simulink model "bell_nexus_4ex_model"  (R2024a)
settings: Solver=ode4  StartTime=0.0  StopTime=simt  FixedStep=st  RelTol=1e-3
values from neighbouring files (symbols this model uses):
  ailer_lim = [-15 20]    [bell_nexus_4ex_params.m]
  B_lat_ext = [B_lat, Bw_lat]    [bell_nexus_4ex.m]
  B_lon_ext = [B_lon, Bw_lon]    [bell_nexus_4ex.m]
  C_lat_ext = [C_lat; eye(1,4)]    [bell_nexus_4ex.m]
  C_lon_ext = [C_lon; eye(2,4)]    [bell_nexus_4ex.m]
  D_lat_ext = blkdiag(D_lat, Tw_lat(1,:))    [bell_nexus_4ex.m]
  D_lon_ext = blkdiag(D_lon, Tw_lon(1:2,:))    [bell_nexus_4ex.m]
  deriv_lag = 0.005    [bell_nexus_4ex.m]    (also in bell_nexus_4ex_params.m = 0.05)
  elev_lim = [-15 22]    [bell_nexus_4ex_params.m]
  elev_pf_tau = 0.7    [bell_nexus_4ex_params.m]
  kd_rudder = 0    [bell_nexus_4ex_params.m]
  ki_rudder = 0    [bell_nexus_4ex_params.m]
  kp_rudder = 0.5    [bell_nexus_4ex_params.m]
  phi_slope = 0    [bell_nexus_4ex.m]
  phi_sp = 0    [bell_nexus_4ex.m]
  phi_st_time = 4    [bell_nexus_4ex.m]
  r_slope = 0    [bell_nexus_4ex.m]
  r_sp = 0    [bell_nexus_4ex.m]
  r_st_time = 4    [bell_nexus_4ex.m]
  rate_lim = 30    [bell_nexus_4ex_params.m]
  rudder_lim = [-25 25]    [bell_nexus_4ex_params.m]
  tau = 0.1    [bell_nexus_4ex_params.m]
  theta_slope = 0    [bell_nexus_4ex.m]
  theta_sp = 0    [bell_nexus_4ex.m]
  theta_st_time = 4    [bell_nexus_4ex.m]
  w_st_time = 4    [bell_nexus_4ex.m]
  wind_lat = [0 0 0]    [bell_nexus_4ex.m]
  wind_lon = [0 0 0]    [bell_nexus_4ex.m]
undefined symbols (not defined in the file or in its folder): A_lat, A_lon, kd_aileron, kd_elevator, ki_aileron, ki_elevator, kp_aileron, kp_elevator, u0
libraries: slpidlib x3, simulink x3
settings Model: Creator=pries  LastModifiedBy=pries
settings RTWCC: GPUComputeCapability=3.5

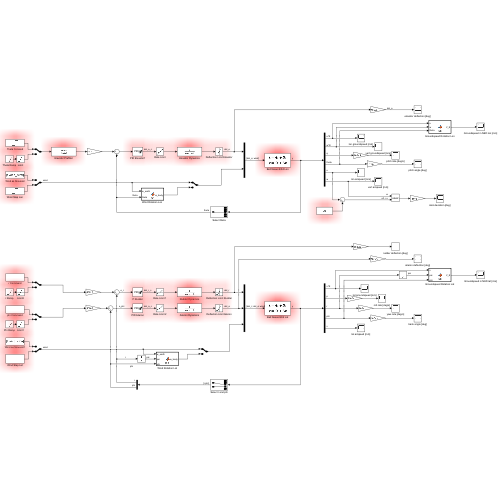
[thumbnail: Simulink's stored preview of the top-level diagram]
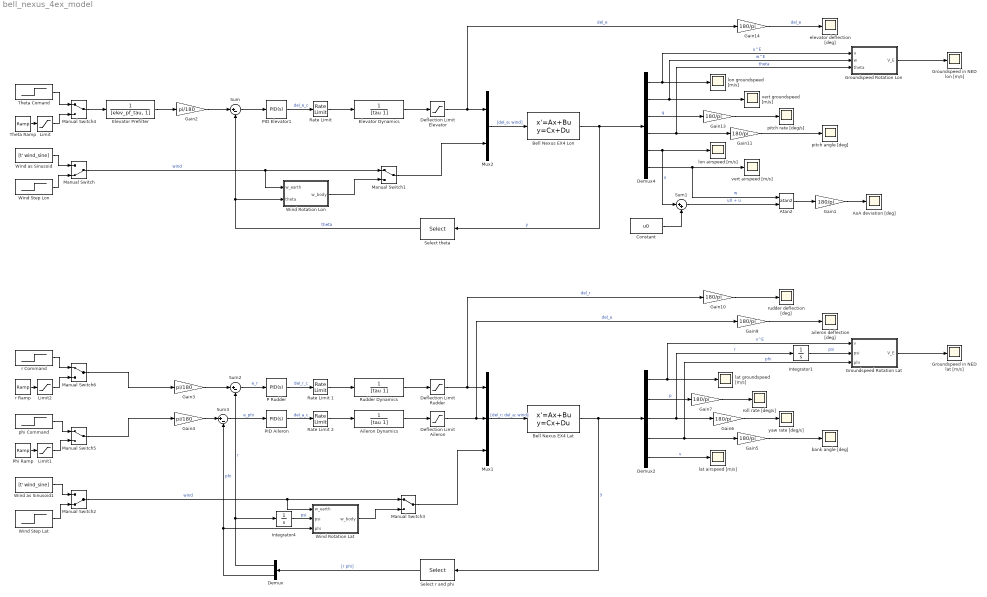
== system bell_nexus_4ex_model ==
  Aileron Dynamics : TransferFcn  Denominator=[tau 1]
  AoA deviation [deg] : Scope
  Atan2 : Trigonometry  Operator=atan2
  Bell Nexus EX4 Lat : StateSpace  A=A_lat  B=B_lat_ext  C=C_lat_ext  D=D_lat_ext  InitialCondition=0  ParameterTunability=Optimized
  Bell Nexus EX4 Lon : StateSpace  A=A_lon  B=B_lon_ext  C=C_lon_ext  D=D_lon_ext  InitialCondition=0
  Constant : Constant  Value=u0
  Deflection Limit Aileron : Saturate  UpperLimit=ailer_lim(2)*pi/180  LowerLimit=ailer_lim(1)*pi/180
  Deflection Limit Elevator : Saturate  UpperLimit=elev_lim(2)*pi/180  LowerLimit=elev_lim(1)*pi/180
  Deflection Limit Rudder : Saturate  UpperLimit=rudder_lim(2)*pi/180  LowerLimit=rudder_lim(1)*pi/180
  Demux : Demux  Outputs=2
  Demux2 : Demux  Outputs=5
  Demux4 : Demux  Outputs=6
  Elevator Dynamics : TransferFcn  Denominator=[tau 1]
  Elevator Prefilter : TransferFcn  Denominator=[elev_pf_tau, 1]
  Gain{1,5..7,9..11,13..14} (9 alike) : Gain  Gain=180/pi
  Gain2 : Gain  Gain=pi/180
  Gain3 : Gain  Gain=pi/180
  Gain4 : Gain  Gain=pi/180
  Groundspeed Rotation Lat : MATLAB Function  TreatAsAtomicUnit=on
  Groundspeed Rotation Lon : MATLAB Function  TreatAsAtomicUnit=on
  Groundspeed in NED lat [m/s] : Scope
  Groundspeed in NED lon [m/s] : Scope
  Integrator1 : Integrator
  Integrator4 : Integrator
  Limit : Saturate  UpperLimit=abs(theta_sp)  LowerLimit=-abs(theta_sp)
  Limit1 : Saturate  UpperLimit=abs(phi_sp)  LowerLimit=-abs(phi_sp)  LinearizeAsGain=off
  Limit2 : Saturate  UpperLimit=abs(r_sp)  LowerLimit=-abs(r_sp)  LinearizeAsGain=off
  Manual Switch : ManualSwitch  CurrentSetting=0
  Manual Switch{1,3..6} (5 alike) : ManualSwitch
  Manual Switch2 : ManualSwitch  CurrentSetting=0
  Mux1 : Mux  Inputs=3
  Mux2 : Mux  Inputs=2
  P Rudder : slpidlib/PID Controller  Controller=PID  Form=Parallel  TimeDomain=Continuous-time  UseExternalTs=off  SampleTime=-1  IntegratorMethod=Forward Euler  FilterMethod=Forward Euler  ControllerParametersSource=internal  P=kp_rudder  I=ki_rudder  UseKiTs=off  D=kd_rudder  UseExternalDerivativeSource=off  N=1/deriv_lag  UseFilter=on  TunerSelectOption=Transfer Function Based (PID Tuner App)  InitialConditionSource=internal  InitialConditionForIntegrator=0  InitialConditionForFilter=0  DifferentiatorICPrevScaledInput=0  ExternalReset=none  TrackingMode=off  Kt=1  LimitOutput=on  SatLimitsSource=internal  UpperSaturationLimit=rudder_lim(2)*pi/180  LowerSaturationLimit=rudder_lim(1)*pi/180  LinearizeAsGain=on  AntiWindupMode=back-calculation  Kb=1  LimitIntegrator=off  UpperIntegratorSaturationLimit=inf  LowerIntegratorSaturationLimit=-inf  POutMin=[]  POutMax=[]  IOutMin=[]  IOutMax=[]  DOutMin=[]  DOutMax=[]  NOutMin=[]  NOutMax=[]  SumOutMin=[]  SumOutMax=[]  SaturationOutMin=[]  SaturationOutMax=[]  PParamMin=[]  PParamMax=[]  IParamMin=[]  IParamMax=[]  DParamMin=[]  DParamMax=[]  NParamMin=[]  NParamMax=[]  KbParamMin=[]  KbParamMax=[]  KtParamMin=[]  KtParamMax=[]  KbOutMin=[]  KbOutMax=[]  KtOutMin=[]  KtOutMax=[]  IntegratorOutMin=[]  IntegratorOutMax=[]  FilterOutMin=[]  FilterOutMax=[]  SumI1OutMin=[]  SumI1OutMax=[]  SumI2OutMin=[]  SumI2OutMax=[]  SumI3OutMin=[]  SumI3OutMax=[]  SumI4OutMin=[]  SumI4OutMax=[]  SumDOutMin=[]  SumDOutMax=[]  DifferentiatorOutMin=[]  DifferentiatorOutMax=[]  FilterDiffOutCoefMin=[]  FilterDiffOutCoefMax=[]  ReciprocalOutMin=[]  ReciprocalOutMax=[]  SumDenOutMin=[]  SumDenOutMax=[]  SumNumOutMin=[]  SumNumOutMax=[]  DivideOutMin=[]  DivideOutMax=[]  UdiffTsProdOutMin=[]  UdiffTsProdOutMax=[]  NTsProdOutMin=[]  NTsProdOutMax=[]  UintegralTsProdOutMin=[]  UintegralTsProdOutMax=[]  UngainTsProdOutMin=[]  UngainTsProdOutMax=[]  ClampingZeroOutDataTypeStr=Inherit: Inherit via back propagation  ClampingZeroOutMin=[]  ClampingZeroOutMax=[]  FilterDenConstantOutDataTypeStr=Inherit: Inherit via back propagation  FilterDenConstantOutMin=[]  FilterDenConstantOutMax=[]  PCopyOutDataTypeStr=Inherit: Inherit via back propagation  PCopyOutMin=[]  PCopyOutMax=[]  NCopyOutDataTypeStr=Inherit: Inherit via back propagation  NCopyOutMin=[]  NCopyOutMax=[]  IntegratorContinuousStateAttributes=''  IntegratorStateMustResolveToSignalObject=off  IntegratorRTWStateStorageClass=Auto  FilterContinuousStateAttributes=''  FilterStateMustResolveToSignalObject=off  FilterRTWStateStorageClass=Auto  ParallelPVariant=InternalParameters  IdealPVariant=Disabled  IVariant=InternalParameters  DVariant=InternalParameters  IntegratorVariant=Continuous  SatVariant=Enabled  AWVariant=BackCalculation  PCopyVariant=Disabled  TRVariant=Disabled  FdbkBlocksVariant=Forward  IdealPFdbkVariant=Disabled  SatFdbkVariant=Disabled  DerivativeFilterVariant=ContFilter  NVariant=InternalParameters  NCopyVariant=Disabled  FilterICVariant=InternalICsFilter  IntegratorICVariant=InternalICs  ExternalResetVariant=Disabled  TRSumVariant=Passthrough  SumFdbkVariant=Disabled  SumVariant=Sum_PID  TsampFilterVariant=InternalTs  TsampNgainVariant=Passthrough  TsampIntegralVariant=Disabled_SignalSpec  ExternalSaturationOutDataTypeStr=Inherit: Same as second input  DerivativeSourceVariant=ErrorSignal
  PID Aileron : slpidlib/PID Controller  Controller=PID  Form=Parallel  TimeDomain=Continuous-time  UseExternalTs=off  SampleTime=-1  IntegratorMethod=Forward Euler  FilterMethod=Forward Euler  ControllerParametersSource=internal  P=kp_aileron  I=ki_aileron  UseKiTs=off  D=kd_aileron  UseExternalDerivativeSource=off  N=1/deriv_lag  UseFilter=on  TunerSelectOption=Transfer Function Based (PID Tuner App)  InitialConditionSource=internal  InitialConditionForIntegrator=0  InitialConditionForFilter=0  DifferentiatorICPrevScaledInput=0  ExternalReset=none  TrackingMode=off  Kt=1  LimitOutput=on  SatLimitsSource=internal  UpperSaturationLimit=ailer_lim(2)*pi/180  LowerSaturationLimit=ailer_lim(1)*pi/180  LinearizeAsGain=on  AntiWindupMode=none  Kb=1  LimitIntegrator=off  UpperIntegratorSaturationLimit=inf  LowerIntegratorSaturationLimit=-inf  POutMin=[]  POutMax=[]  IOutMin=[]  IOutMax=[]  DOutMin=[]  DOutMax=[]  NOutMin=[]  NOutMax=[]  SumOutMin=[]  SumOutMax=[]  SaturationOutMin=[]  SaturationOutMax=[]  PParamMin=[]  PParamMax=[]  IParamMin=[]  IParamMax=[]  DParamMin=[]  DParamMax=[]  NParamMin=[]  NParamMax=[]  KbParamMin=[]  KbParamMax=[]  KtParamMin=[]  KtParamMax=[]  KbOutMin=[]  KbOutMax=[]  KtOutMin=[]  KtOutMax=[]  IntegratorOutMin=[]  IntegratorOutMax=[]  FilterOutMin=[]  FilterOutMax=[]  SumI1OutMin=[]  SumI1OutMax=[]  SumI2OutMin=[]  SumI2OutMax=[]  SumI3OutMin=[]  SumI3OutMax=[]  SumI4OutMin=[]  SumI4OutMax=[]  SumDOutMin=[]  SumDOutMax=[]  DifferentiatorOutMin=[]  DifferentiatorOutMax=[]  FilterDiffOutCoefMin=[]  FilterDiffOutCoefMax=[]  ReciprocalOutMin=[]  ReciprocalOutMax=[]  SumDenOutMin=[]  SumDenOutMax=[]  SumNumOutMin=[]  SumNumOutMax=[]  DivideOutMin=[]  DivideOutMax=[]  UdiffTsProdOutMin=[]  UdiffTsProdOutMax=[]  NTsProdOutMin=[]  NTsProdOutMax=[]  UintegralTsProdOutMin=[]  UintegralTsProdOutMax=[]  UngainTsProdOutMin=[]  UngainTsProdOutMax=[]  ClampingZeroOutDataTypeStr=Inherit: Inherit via back propagation  ClampingZeroOutMin=[]  ClampingZeroOutMax=[]  FilterDenConstantOutDataTypeStr=Inherit: Inherit via back propagation  FilterDenConstantOutMin=[]  FilterDenConstantOutMax=[]  PCopyOutDataTypeStr=Inherit: Inherit via back propagation  PCopyOutMin=[]  PCopyOutMax=[]  NCopyOutDataTypeStr=Inherit: Inherit via back propagation  NCopyOutMin=[]  NCopyOutMax=[]  IntegratorContinuousStateAttributes=''  IntegratorStateMustResolveToSignalObject=off  IntegratorRTWStateStorageClass=Auto  FilterContinuousStateAttributes=''  FilterStateMustResolveToSignalObject=off  FilterRTWStateStorageClass=Auto  ParallelPVariant=InternalParameters  IdealPVariant=Disabled  IVariant=InternalParameters  DVariant=InternalParameters  IntegratorVariant=Continuous  SatVariant=Enabled  AWVariant=Passthrough  PCopyVariant=Disabled  TRVariant=Disabled  FdbkBlocksVariant=Forward  IdealPFdbkVariant=Disabled  SatFdbkVariant=Disabled  DerivativeFilterVariant=ContFilter  NVariant=InternalParameters  NCopyVariant=Disabled  FilterICVariant=InternalICsFilter  IntegratorICVariant=InternalICs  ExternalResetVariant=Disabled  TRSumVariant=Passthrough  SumFdbkVariant=Disabled  SumVariant=Sum_PID  TsampFilterVariant=InternalTs  TsampNgainVariant=Passthrough  TsampIntegralVariant=Disabled_SignalSpec  ExternalSaturationOutDataTypeStr=Inherit: Same as second input  DerivativeSourceVariant=ErrorSignal
  PID Elevator1 : slpidlib/PID Controller  Controller=PID  Form=Parallel  TimeDomain=Continuous-time  UseExternalTs=off  SampleTime=-1  IntegratorMethod=Forward Euler  FilterMethod=Forward Euler  ControllerParametersSource=internal  P=kp_elevator  I=ki_elevator  UseKiTs=off  D=kd_elevator  UseExternalDerivativeSource=off  N=1/deriv_lag  UseFilter=on  TunerSelectOption=Transfer Function Based (PID Tuner App)  InitialConditionSource=internal  InitialConditionForIntegrator=0  InitialConditionForFilter=0  DifferentiatorICPrevScaledInput=0  ExternalReset=none  TrackingMode=off  Kt=1  LimitOutput=on  SatLimitsSource=internal  UpperSaturationLimit=elev_lim(2)*pi/180  LowerSaturationLimit=elev_lim(1)*pi/180  LinearizeAsGain=on  AntiWindupMode=back-calculation  Kb=1  LimitIntegrator=off  UpperIntegratorSaturationLimit=inf  LowerIntegratorSaturationLimit=-inf  POutMin=[]  POutMax=[]  IOutMin=[]  IOutMax=[]  DOutMin=[]  DOutMax=[]  NOutMin=[]  NOutMax=[]  SumOutMin=[]  SumOutMax=[]  SaturationOutMin=[]  SaturationOutMax=[]  PParamMin=[]  PParamMax=[]  IParamMin=[]  IParamMax=[]  DParamMin=[]  DParamMax=[]  NParamMin=[]  NParamMax=[]  KbParamMin=[]  KbParamMax=[]  KtParamMin=[]  KtParamMax=[]  KbOutMin=[]  KbOutMax=[]  KtOutMin=[]  KtOutMax=[]  IntegratorOutMin=[]  IntegratorOutMax=[]  FilterOutMin=[]  FilterOutMax=[]  SumI1OutMin=[]  SumI1OutMax=[]  SumI2OutMin=[]  SumI2OutMax=[]  SumI3OutMin=[]  SumI3OutMax=[]  SumI4OutMin=[]  SumI4OutMax=[]  SumDOutMin=[]  SumDOutMax=[]  DifferentiatorOutMin=[]  DifferentiatorOutMax=[]  FilterDiffOutCoefMin=[]  FilterDiffOutCoefMax=[]  ReciprocalOutMin=[]  ReciprocalOutMax=[]  SumDenOutMin=[]  SumDenOutMax=[]  SumNumOutMin=[]  SumNumOutMax=[]  DivideOutMin=[]  DivideOutMax=[]  UdiffTsProdOutMin=[]  UdiffTsProdOutMax=[]  NTsProdOutMin=[]  NTsProdOutMax=[]  UintegralTsProdOutMin=[]  UintegralTsProdOutMax=[]  UngainTsProdOutMin=[]  UngainTsProdOutMax=[]  ClampingZeroOutDataTypeStr=Inherit: Inherit via back propagation  ClampingZeroOutMin=[]  ClampingZeroOutMax=[]  FilterDenConstantOutDataTypeStr=Inherit: Inherit via back propagation  FilterDenConstantOutMin=[]  FilterDenConstantOutMax=[]  PCopyOutDataTypeStr=Inherit: Inherit via back propagation  PCopyOutMin=[]  PCopyOutMax=[]  NCopyOutDataTypeStr=Inherit: Inherit via back propagation  NCopyOutMin=[]  NCopyOutMax=[]  IntegratorContinuousStateAttributes=''  IntegratorStateMustResolveToSignalObject=off  IntegratorRTWStateStorageClass=Auto  FilterContinuousStateAttributes=''  FilterStateMustResolveToSignalObject=off  FilterRTWStateStorageClass=Auto  ParallelPVariant=InternalParameters  IdealPVariant=Disabled  IVariant=InternalParameters  DVariant=InternalParameters  IntegratorVariant=Continuous  SatVariant=Enabled  AWVariant=BackCalculation  PCopyVariant=Disabled  TRVariant=Disabled  FdbkBlocksVariant=Forward  IdealPFdbkVariant=Disabled  SatFdbkVariant=Disabled  DerivativeFilterVariant=ContFilter  NVariant=InternalParameters  NCopyVariant=Disabled  FilterICVariant=InternalICsFilter  IntegratorICVariant=InternalICs  ExternalResetVariant=Disabled  TRSumVariant=Passthrough  SumFdbkVariant=Disabled  SumVariant=Sum_PID  TsampFilterVariant=InternalTs  TsampNgainVariant=Passthrough  TsampIntegralVariant=Disabled_SignalSpec  ExternalSaturationOutDataTypeStr=Inherit: Same as second input  DerivativeSourceVariant=ErrorSignal
  Phi Ramp : simulink/Sources/Ramp  slope=phi_slope  start=phi_st_time  InitialOutput=0
  Rate Limit : RateLimiter  RisingSlewLimit=rate_lim*pi/180  FallingSlewLimit=-rate_lim*pi/180  SampleTimeMode=inherited
  Rate Limit 1 : RateLimiter  RisingSlewLimit=rate_lim*pi/180  FallingSlewLimit=-rate_lim*pi/180  SampleTimeMode=inherited
  Rate Limit 2 : RateLimiter  RisingSlewLimit=rate_lim*pi/180  FallingSlewLimit=-rate_lim*pi/180  SampleTimeMode=inherited
  Rudder Dynamics : TransferFcn  Denominator=[tau 1]
  Select r and phi : Selector  InputPortWidth=5  IndexOptions=Index vector (dialog)  Indices=[3, 4]  OutputSizes=1
  Select theta : Selector  InputPortWidth=6  IndexOptions=Index vector (dialog)  Indices=[4]  OutputSizes=1
  Sum : Sum  Inputs=|+-
  Sum1 : Sum  Inputs=|++
  Sum2 : Sum  Inputs=|+-
  Sum3 : Sum  Inputs=|+-
  Theta Comand : Step  Time=theta_st_time  After=theta_sp  SampleTime=0
  Theta Ramp : simulink/Sources/Ramp  slope=theta_slope  start=theta_st_time  InitialOutput=0
  Wind Rotation Lat : MATLAB Function  TreatAsAtomicUnit=on
  "Wind Rotation Lon " : MATLAB Function  TreatAsAtomicUnit=on
  Wind Step Lat : Step  Time=w_st_time  Before=[0 0 0]  After=wind_lat  SampleTime=0
  Wind Step Lon : Step  Time=w_st_time  Before=[0 0 0]  After=wind_lon  SampleTime=0
  Wind as Sinusoid : FromWorkspace  VariableName=[t' wind_sine]
  Wind as Sinusoid1 : FromWorkspace  VariableName=[t' wind_sine]
  aileron deflection [deg] : Scope
  bank angle [deg] : Scope
  elevator deflection [deg] : Scope
  lat airspeed [m/s] : Scope
  lat groundspeed [m/s] : Scope
  lon airspeed [m/s] : Scope
  lon groundspeed [m/s] : Scope
  phi Command : Step  Time=phi_st_time  After=phi_sp  SampleTime=0
  pitch angle [deg] : Scope
  pitch rate [deg/s] : Scope
  r Command : Step  Time=r_st_time  After=r_sp  SampleTime=0
  r Ramp : simulink/Sources/Ramp  slope=r_slope  start=r_st_time  InitialOutput=0
  roll rate [deg/s] : Scope
  rudder deflection [deg] : Scope
  vert airspeed [m/s] : Scope
  vert groundspeed [m/s] : Scope
  yaw rate [deg/s] : Scope
  wires:
  Bell Nexus EX4 Lon/1 -> Demux4/1, Select theta/1  "y"
  Demux4/1 -> Groundspeed Rotation Lon/1(u), lon groundspeed [m/s]/1  "u^E"
  Demux4/5 -> Sum1/1, lon airspeed [m/s]/1  "u"
  Demux4/6 -> Atan2/1, vert airspeed [m/s]/1  "w"
  Gain13/1 -> pitch rate [deg/s]/1
  Gain11/1 -> pitch angle [deg]/1
  Demux4/2 -> Groundspeed Rotation Lon/2(w), vert groundspeed [m/s]/1  "w^E"
  Demux4/3 -> Gain13/1  "q"
  Demux4/4 -> Groundspeed Rotation Lon/3(theta), Gain11/1  "theta"
  Select theta/1 -> "Wind Rotation Lon "/2(theta), Sum/2  "theta"
  Elevator Prefilter/1 -> Gain2/1
  Gain2/1 -> Sum/1
  Sum/1 -> PID Elevator1/1
  PID Elevator1/1 -> Rate Limit/1  "del_e_c"
  Rate Limit/1 -> Elevator Dynamics/1
  Elevator Dynamics/1 -> Deflection Limit Elevator/1
  Mux2/1 -> Bell Nexus EX4 Lon/1  "[del_e; wind]"
  Deflection Limit Elevator/1 -> Gain14/1, Mux2/1  "del_e"
  Wind Step Lon/1 -> Manual Switch/2
  Wind as Sinusoid/1 -> Manual Switch/1
  Manual Switch/1 -> Manual Switch1/1, "Wind Rotation Lon "/1(w_earth)  "wind"
  "Wind Rotation Lon "/1(w_body) -> Manual Switch1/2
  Constant/1 -> Sum1/2
  Sum1/1 -> Atan2/2  "u0 + u"
  Atan2/1 -> Gain1/1
  Gain1/1 -> AoA deviation [deg]/1
  Gain14/1 -> elevator deflection [deg]/1  "del_e"
  Bell Nexus EX4 Lat/1 -> Demux2/1, Select r and phi/1  "y"
  Demux2/5 -> lat airspeed [m/s]/1  "v"
  Demux2/1 -> Groundspeed Rotation Lat/1(v), lat groundspeed [m/s]/1  "v^E"
  Demux2/2 -> Gain7/1  "p"
  Demux2/3 -> Integrator1/1, Gain6/1  "r"
  Demux2/4 -> Groundspeed Rotation Lat/3(phi), Gain5/1  "phi"
  Gain5/1 -> bank angle [deg]/1
  Gain6/1 -> yaw rate [deg/s]/1
  Mux1/1 -> Bell Nexus EX4 Lat/1  "[del_r; del_a; wind]"
  Select r and phi/1 -> Demux/1  "[r phi]"
  Demux/1 -> Integrator4/1, Sum2/2  "r"
  Demux/2 -> Sum3/2, Wind Rotation Lat/3(phi)  "phi"
  Gain3/1 -> Sum2/1
  Gain4/1 -> Sum3/1
  Wind as Sinusoid1/1 -> Manual Switch2/1
  Wind Step Lat/1 -> Manual Switch2/2
  P Rudder/1 -> Rate Limit 1/1  "del_r_c"
  PID Aileron/1 -> Rate Limit 2/1  "del_a_c"
  Rate Limit 1/1 -> Rudder Dynamics/1
  Rate Limit 2/1 -> Aileron Dynamics/1
  Aileron Dynamics/1 -> Deflection Limit Aileron/1
  Rudder Dynamics/1 -> Deflection Limit Rudder/1
  Deflection Limit Rudder/1 -> Gain10/1, Mux1/1  "del_r"
  Deflection Limit Aileron/1 -> Gain9/1, Mux1/2  "del_a"
  Sum2/1 -> P Rudder/1  "e_r"
  Sum3/1 -> PID Aileron/1  "e_phi"
  Manual Switch2/1 -> Manual Switch3/1, Wind Rotation Lat/1(w_earth)  "wind"
  Integrator4/1 -> Wind Rotation Lat/2(psi)  "psi"
  Wind Rotation Lat/1(w_body) -> Manual Switch3/2
  Manual Switch3/1 -> Mux1/3
  Gain10/1 -> rudder deflection [deg]/1
  Gain9/1 -> aileron deflection [deg]/1
  Groundspeed Rotation Lon/1(V_E) -> Groundspeed in NED lon [m/s]/1
  Integrator1/1 -> Groundspeed Rotation Lat/2(psi)  "psi"
  Groundspeed Rotation Lat/1(V_E) -> Groundspeed in NED lat [m/s]/1
  Gain7/1 -> roll rate [deg/s]/1
  Theta Ramp/1 -> Limit/1
  Manual Switch4/1 -> Elevator Prefilter/1
  Limit/1 -> Manual Switch4/2
  Theta Comand/1 -> Manual Switch4/1
  Limit1/1 -> Manual Switch5/2
  Phi Ramp/1 -> Limit1/1
  r Ramp/1 -> Limit2/1
  Limit2/1 -> Manual Switch6/2
  phi Command/1 -> Manual Switch5/1
  Manual Switch5/1 -> Gain4/1
  r Command/1 -> Manual Switch6/1
  Manual Switch6/1 -> Gain3/1
  Manual Switch1/1 -> Mux2/2

== matlab function bell_nexus_4ex_model/Wind Rotation Lat ==
  data: w_earth input; psi input; w_body output; phi input
function w_body = fcn(w_earth, psi, phi)
rot = eul2rotm([-psi 0 -phi]);
w_body = rot*w_earth;

== matlab function bell_nexus_4ex_model/Wind Rotation Lon  ==
  data: w_earth input; w_body output; theta input
function w_body = fcn(w_earth, theta)
rot = eul2rotm([0 -theta 0]);
w_body = rot*w_earth;

== matlab function bell_nexus_4ex_model/Groundspeed Rotation Lon ==
  data: u input; w input; V_E output; theta input
function V_E = fcn(u, w, theta)
rot = eul2rotm([0 theta 0]);
V_E = rot*[u 0 w]';

== matlab function bell_nexus_4ex_model/Groundspeed Rotation Lat ==
  data: v input; psi input; V_E output; phi input
function V_E = fcn(v, psi, phi)
rot = eul2rotm([psi 0 phi]);
V_E = rot*[0 v 0]';
